simulink model "RR_DC_motor"  (R2023a)
settings: Solver=VariableStepAuto  StartTime=0.0  StopTime=15  RelTol=1e-6
values from neighbouring files (symbols this model uses):
  b = 0.1    [main_RR_VR.m]
  dq0 = [0.0 ; 0.0]    [main_RR_VR.m]
  dq0_d = [0.0; 0.0]    [main_RR_VR.m]
  Il = (1/3)*m1*a1^2    (= 1.66666666667)    [main_RR_VR.m]
  Im = 740e-6    (= 0.00074)    [main_RR_VR.m]
  k_mot = 0.23    [main_RR_VR.m]
  K_pid = 5    [main_RR_VR.m]
  L = 50e-6    (= 5e-05)    [main_RR_VR.m]
  q0 = [0.25 ; 0.25]    [main_RR_VR.m]
  q0_d = [pi/2; -pi/2]    [main_RR_VR.m]
  q1_0 = q0(1)    [main_RR_VR.m]
  q2_0 = q0(2)    [main_RR_VR.m]
  R = 0.11    [main_RR_VR.m]
settings Model: Creator=Mathew  LastModifiedBy=rvitt
settings SolverCC: AlgebraicLoopSolver=TrustRegion
settings OptimizationCC: ReuseModelBlockBuffer=off
settings DebuggingCC: UnconnectedInputMsg=warning  UnconnectedOutputMsg=warning  UnconnectedLineMsg=warning  ArithmeticOperatorsInVariantConditions=warning
settings ModelReferenceCC: EnableRefExpFcnMdlSchedulingChecks=on
settings SFSimCC: CustomCodeUndefinedFunction=UseInterfaceOnly

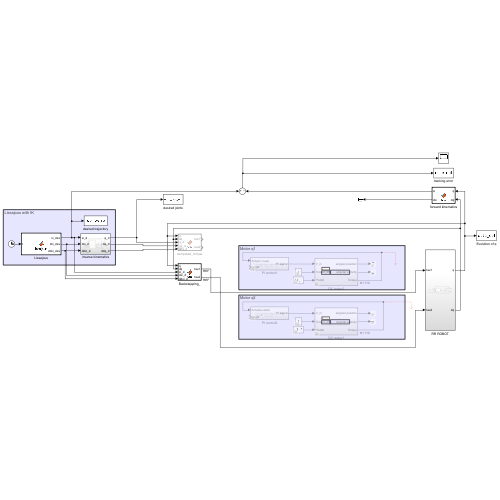
[thumbnail: Simulink's stored preview of the top-level diagram]
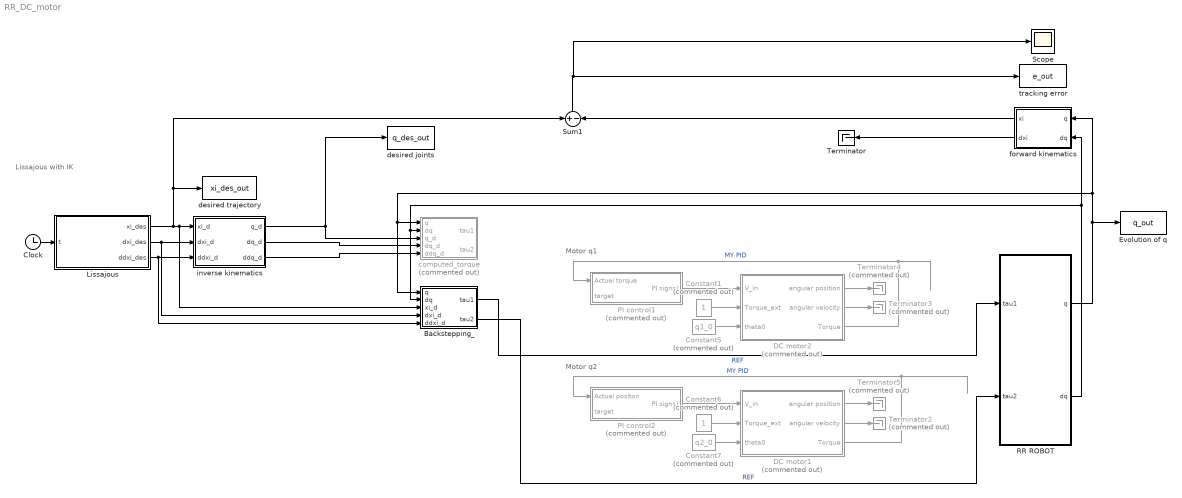
== system RR_DC_motor ==
  note: Lissajous with IK
  note: Motor q1
  note: Motor q2
  Backstepping_ : MATLAB Function  TreatAsAtomicUnit=on
  Clock : Clock
  Constant1 : Constant  Commented=on
  Constant5 : Constant  Commented=on  Value=q1_0
  Constant6 : Constant  Commented=on
  Constant7 : Constant  Commented=on  Value=q2_0
  DC motor1 : Subsystem  Commented=on
  DC motor2 : Subsystem  Commented=on
  Evolution of q : ToWorkspace  VariableName=q_out  SaveFormat=Timeseries  SampleTime=-1
  Lissajous : MATLAB Function  TreatAsAtomicUnit=on
  PI control1 : Subsystem  Commented=on
  PI control2 : Subsystem  Commented=on
  RR ROBOT : Subsystem
  Scope : Scope
  Sum1 : Sum  Inputs=+-
  Terminator : Terminator
  Terminator{2..5} (4 alike) : Terminator  Commented=on
  computed_torque : MATLAB Function  Commented=on  TreatAsAtomicUnit=on
  desired joints : ToWorkspace  VariableName=q_des_out  SaveFormat=Timeseries  SampleTime=-1
  desired trajectory : ToWorkspace  VariableName=xi_des_out  SaveFormat=Timeseries  SampleTime=-1
  forward kinematics : MATLAB Function  TreatAsAtomicUnit=on
  inverse kinematics : Subsystem
  tracking error : ToWorkspace  VariableName=e_out  SaveFormat=Timeseries  SampleTime=-1
  wires:
  RR ROBOT/1(q) -> Backstepping_/1(q), computed_torque/1(q), forward kinematics/1(q), Evolution of q/1
  RR ROBOT/2(dq) -> Backstepping_/2(dq), computed_torque/2(dq), forward kinematics/2(dq)
  inverse kinematics/1(q_d) -> computed_torque/3(q_d), desired joints/1
  Clock/1 -> Lissajous/1(t)
  Lissajous/2(dxi_des) -> Backstepping_/4(dxi_d), inverse kinematics/2(dxi_d)
  Lissajous/3(ddxi_des) -> Backstepping_/5(ddxi_d), inverse kinematics/3(ddxi_d)
  Lissajous/1(xi_des) -> Sum1/1, desired trajectory/1, Backstepping_/3(xi_d), inverse kinematics/1(xi_d)
  Sum1/1 -> Scope/1, tracking error/1
  forward kinematics/2(dxi) -> Terminator/1
  forward kinematics/1(xi) -> Sum1/2
  inverse kinematics/2(dq_d) -> computed_torque/4(dq_d)
  inverse kinematics/3(ddq_d) -> computed_torque/5(ddq_d)
  PI control1/1(PI signal) -> DC motor2/1(V_in)
  DC motor2/1(angular position) -> Terminator4/1
  DC motor2/2(angular velocity) -> Terminator3/1
  Constant1/1 -> DC motor2/2(Torque_ext)
  Constant5/1 -> DC motor2/3(theta0)
  DC motor2/3(Torque) -> PI control1/1(Actual torque)  "MY PID"
  DC motor1/3(Torque) -> PI control2/1(Actual positon)  "MY PID"
  Constant7/1 -> DC motor1/3(theta0)
  Constant6/1 -> DC motor1/2(Torque_ext)
  DC motor1/2(angular velocity) -> Terminator2/1
  DC motor1/1(angular position) -> Terminator5/1
  PI control2/1(PI signal) -> DC motor1/1(V_in)
  Backstepping_/1(tau1) -> RR ROBOT/1(tau1)  "REF"
  Backstepping_/2(tau2) -> RR ROBOT/2(tau2)  "REF"

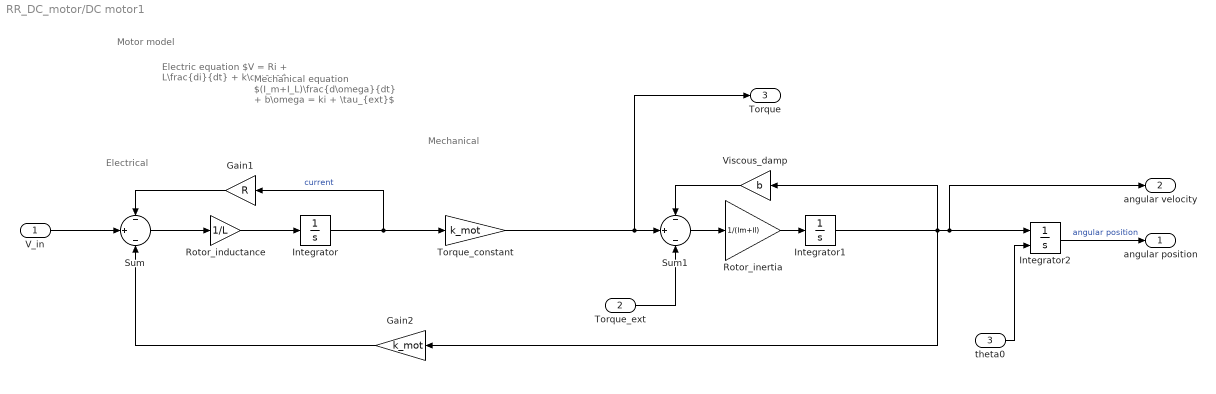
== system RR_DC_motor/DC motor1 ==
  note: Electric equation
      | $V = Ri + L\frac{di}{dt} + k\omega$
  note: Mechanical equation
      | $(I_m+I_L)\frac{d\omega}{dt} + b\omega = ki + \tau_{ext}$
  note: Motor model
  note: Electrical
  note: Mechanical
  V_in : Inport
  Torque_ext : Inport  Port=2
  theta0 : Inport  Port=3
  Gain1 : Gain  Gain=R
  Gain2 : Gain  Gain=k_mot
  Integrator : Integrator
  Integrator1 : Integrator
  Integrator2 : Integrator  InitialConditionSource=external
  Rotor_inductance : Gain  Gain=1/L
  Rotor_inertia : Gain  Gain=1/(Im+Il)
  Sum : Sum  Inputs=-|+|-
  Sum1 : Sum  Inputs=-|+|-
  Torque_constant : Gain  Gain=k_mot
  Viscous_damp : Gain  Gain=b
  angular position : Outport
  angular velocity : Outport  Port=2
  Torque : Outport  Port=3
  wires:
  theta0/1 -> Integrator2/2
  Integrator1/1 -> Gain2/1, Integrator2/1, angular velocity/1, Viscous_damp/1
  Torque_constant/1 -> Sum1/2, Torque/1
  Integrator2/1 -> angular position/1  "angular position"
  Gain2/1 -> Sum/3
  Gain1/1 -> Sum/1
  Rotor_inertia/1 -> Integrator1/1
  V_in/1 -> Sum/2
  Rotor_inductance/1 -> Integrator/1
  Sum1/1 -> Rotor_inertia/1
  Torque_ext/1 -> Sum1/3
  Viscous_damp/1 -> Sum1/1
  Integrator/1 -> Torque_constant/1, Gain1/1  "current"
  Sum/1 -> Rotor_inductance/1

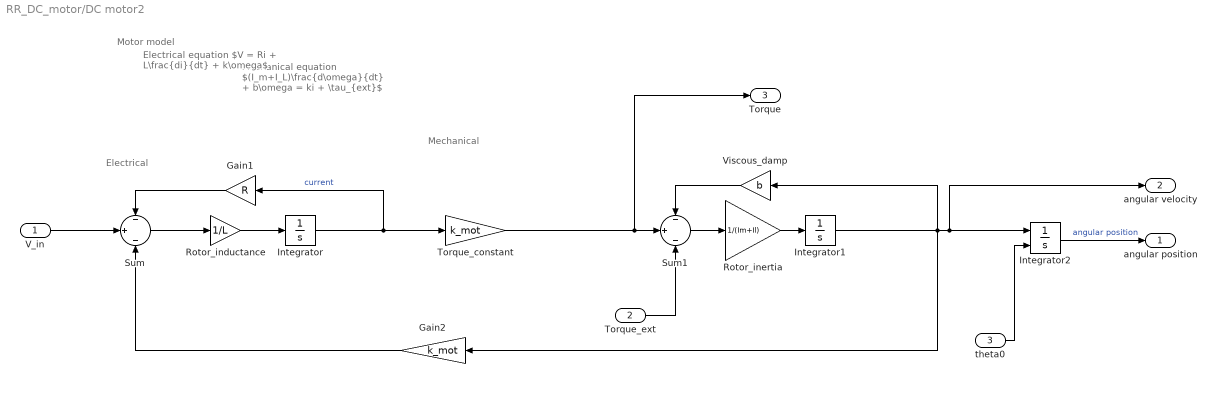
== system RR_DC_motor/DC motor2 ==
  note: Mechanical
  note: Electrical
  note: Motor model
  note: Mechanical equation
      | $(I_m+I_L)\frac{d\omega}{dt} + b\omega = ki + \tau_{ext}$
  note: Electrical equation
      | $V = Ri + L\frac{di}{dt} + k\omega$
  V_in : Inport
  Torque_ext : Inport  Port=2
  theta0 : Inport  Port=3
  Gain1 : Gain  Gain=R
  Gain2 : Gain  Gain=k_mot
  Integrator : Integrator
  Integrator1 : Integrator
  Integrator2 : Integrator  InitialConditionSource=external
  Rotor_inductance : Gain  Gain=1/L
  Rotor_inertia : Gain  Gain=1/(Im+Il)
  Sum : Sum  Inputs=-|+|-
  Sum1 : Sum  Inputs=-|+|-
  Torque_constant : Gain  Gain=k_mot
  Viscous_damp : Gain  Gain=b
  angular position : Outport
  angular velocity : Outport  Port=2
  Torque : Outport  Port=3
  wires:
  Sum/1 -> Rotor_inductance/1
  Integrator/1 -> Gain1/1, Torque_constant/1  "current"
  Viscous_damp/1 -> Sum1/1
  Torque_ext/1 -> Sum1/3
  Sum1/1 -> Rotor_inertia/1
  Rotor_inductance/1 -> Integrator/1
  V_in/1 -> Sum/2
  Rotor_inertia/1 -> Integrator1/1
  Gain1/1 -> Sum/1
  Gain2/1 -> Sum/3
  Integrator2/1 -> angular position/1  "angular position"
  Torque_constant/1 -> Torque/1, Sum1/2
  Integrator1/1 -> Viscous_damp/1, angular velocity/1, Integrator2/1, Gain2/1
  theta0/1 -> Integrator2/2

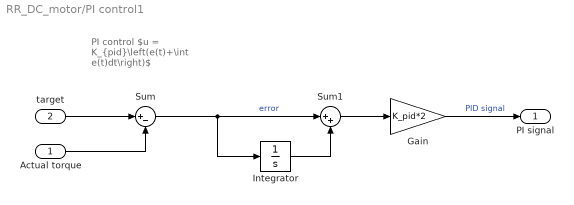
== system RR_DC_motor/PI control1 ==
  note: PI control
      | $u = K_{pid}\left(e(t)+\int e(t)dt\right)$
  Actual torque : Inport
  target : Inport  Port=2
  Gain : Gain  Gain=K_pid*2
  Integrator : Integrator
  Sum : Sum  Inputs=|+-
  Sum1 : Sum  Inputs=|++
  PI signal : Outport
  wires:
  Actual torque/1 -> Sum/2
  Sum1/1 -> Gain/1
  Gain/1 -> PI signal/1  "PID signal"
  Sum/1 -> Sum1/1, Integrator/1  "error"
  target/1 -> Sum/1
  Integrator/1 -> Sum1/2

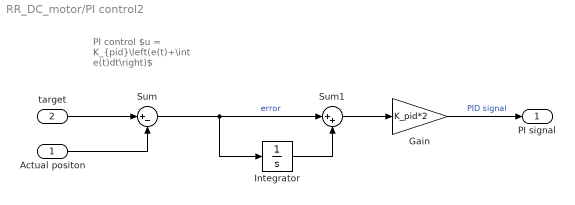
== system RR_DC_motor/PI control2 ==
  note: PI control
      | $u = K_{pid}\left(e(t)+\int e(t)dt\right)$
  Actual positon : Inport
  target : Inport  Port=2
  Gain : Gain  Gain=K_pid*2
  Integrator : Integrator
  Sum : Sum  Inputs=|+-
  Sum1 : Sum  Inputs=|++
  PI signal : Outport
  wires:
  Integrator/1 -> Sum1/2
  target/1 -> Sum/1
  Sum/1 -> Integrator/1, Sum1/1  "error"
  Gain/1 -> PI signal/1  "PID signal"
  Sum1/1 -> Gain/1
  Actual positon/1 -> Sum/2

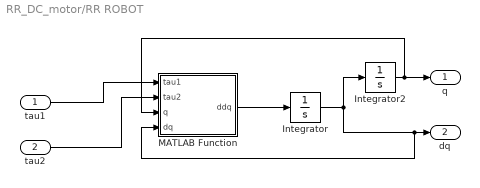
== system RR_DC_motor/RR ROBOT ==
  tau1 : Inport
  tau2 : Inport  Port=2
  Integrator : Integrator  InitialCondition=dq0
  Integrator2 : Integrator  InitialCondition=q0
  MATLAB Function : MATLAB Function  TreatAsAtomicUnit=on
  q : Outport  PortDimensions=[2,1]
  dq : Outport  Port=2  PortDimensions=[2,1]
  wires:
  tau1/1 -> MATLAB Function/1(tau1)
  MATLAB Function/1(ddq) -> Integrator/1
  Integrator/1 -> Integrator2/1, MATLAB Function/4(dq), dq/1
  Integrator2/1 -> MATLAB Function/3(q), q/1
  tau2/1 -> MATLAB Function/2(tau2)

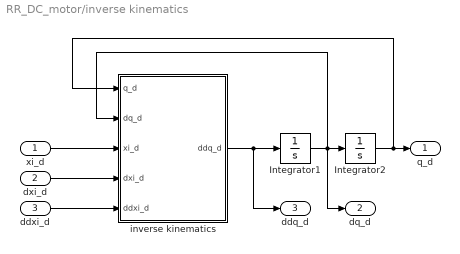
== system RR_DC_motor/inverse kinematics ==
  xi_d : Inport
  dxi_d : Inport  Port=2
  ddxi_d : Inport  Port=3
  Integrator1 : Integrator  InitialCondition=dq0_d
  Integrator2 : Integrator  InitialCondition=q0_d
  inverse kinematics : MATLAB Function  TreatAsAtomicUnit=on
  q_d : Outport  PortDimensions=[2,1]
  dq_d : Outport  Port=2  PortDimensions=[2,1]
  ddq_d : Outport  Port=3  PortDimensions=[2,1]
  wires:
  inverse kinematics/1(ddq_d) -> Integrator1/1, ddq_d/1
  Integrator2/1 -> inverse kinematics/1(q_d), q_d/1
  ddxi_d/1 -> inverse kinematics/5(ddxi_d)
  dxi_d/1 -> inverse kinematics/4(dxi_d)
  xi_d/1 -> inverse kinematics/3(xi_d)
  Integrator1/1 -> inverse kinematics/2(dq_d), dq_d/1, Integrator2/1

== matlab function RR_DC_motor/computed_torque ==
  data: q input; tau1 output; dq input; q_d input; dq_d input; ddq_d input; params parameter; tau2 output
function [tau1, tau2]  = fcn(q, dq, q_d, dq_d, ddq_d, params)

% robot matrix
M = get_M(q,params);
C = get_C(q,dq,params);
G = get_G(q, params);

% errors computation
e = q_d - q;
de = dq_d - dq;

% gains
kp = 5;
kv = 3;

% computed torque
tau = M*(ddq_d + kv*de + kp*e) + C*dq + G;

% robustness
A = [zeros(2,2) eye(2,2);...
    -kp*eye(2,2) -kv*eye(2,2)];

B = [zeros(2,2); eye(2,2)];

coder.extrinsic('lyap');
P = zeros(4,4);
P = lyap(A', eye(4,4));

x = [e; de];

w = B'*P*x;
rho = 10;
eps = 0.001;

delta = rho*w / (sqrt(w'*w + eps));

tau = tau + M*delta;

tau1 = tau(1);
tau2 = tau(2);

== matlab function RR_DC_motor/RR ROBOT/MATLAB Function ==
  data: tau1 input; tau2 input; ddq output; q input; dq input; params parameter
function ddq  = fcn(tau1, tau2, q, dq, params)

% get the matrix for the model
M = get_M(q,params);
C = get_C(q,dq,params);
G = get_G(q, params);

% create tau vector
tau = [tau1; tau2];

% inversion of dinamic equations (M def+)
ddq = inv(M)*(tau-C*dq-G);

== matlab function RR_DC_motor/Backstepping_ ==
  data: q input; tau1 output; dq input; xi_d input; dxi_d input; ddxi_d input; params parameter; tau2 output
function [tau1, tau2]  = fcn(q, dq, xi_d, dxi_d, ddxi_d, params)

% uncertanties


% robot matrix
M = get_M(q,params);
C = get_C(q,dq,params);
G = get_G(q, params);

% get end effector position
[xi, dxi] = RR_forward_kinematics(q,dq,params);

% errors computation
e = xi_d - xi;
de = dxi_d - dxi;

% backstepping
J = get_J(q,params);
pinv_J = pinv(J);
lambda = 1;
dq_r = pinv_J * (dxi_d + lambda*e);
kd = 1;

% dynamics
s = dq_r - dq;
J_dot = get_J_dot(q, dq, params);
ddq_r = pinv_J * (ddxi_d - J_dot*dq_r + lambda*de);

% control signal
tau = M*ddq_r + C*dq_r + G + kd*s + J'*e;

tau1 = tau(1);
tau2 = tau(2);

== matlab function RR_DC_motor/Lissajous ==
  data: t input; xi_des output size=[2,1]; dxi_des output size=[2,1]; ddxi_des output size=[2,1]; par_traj parameter
function [xi_des, dxi_des, ddxi_des] = lissajous(t, par_traj)

A = par_traj.A;
B = par_traj.B;
a = par_traj.a;
b = par_traj.b;
d = par_traj.d;
xi0 = par_traj.xi0;

xi_des = [A*sin(a*t+d); B*sin(b*t)] + xi0;
dxi_des = [A*a*cos(a*t+d); B*b*cos(b*t)];
ddxi_des = [-A*a^2*sin(a*t+d); -B*b^2*sin(b*t)];

== matlab function RR_DC_motor/inverse kinematics/inverse kinematics ==
  data: q_d input; dq_d input; xi_d input; dxi_d input; ddxi_d input; ddq_d output; params parameter
function ddq_d = fcn(q_d, dq_d, xi_d, dxi_d, ddxi_d, params)

% jacobian
J = get_J(q_d, params);
% jacobian derivative
J_dot = get_J_dot(q_d, dq_d, params);
% pseudoinverse
pinv_J = pinv(J);
% forward kinematics
[xi_curr, dxi_curr] = RR_forward_kinematics(q_d, dq_d, params);

% second order CLIK
Kp = 100;
Kv = 30;
ddq_d = pinv_J * (ddxi_d - J_dot * dq_d + Kv*(dxi_d-dxi_curr) + Kp*(xi_d-xi_curr));

== matlab function RR_DC_motor/forward kinematics ==
  data: q input; xi output; dq input; params parameter; dxi output
function [xi, dxi] = fcn(q, dq, params)

[xi, dxi] = RR_forward_kinematics(q, dq, params);

end
